simulink model "MagLevTbx_MagSens_v43_Block"  (R2025b)
settings: Solver=FixedStepDiscrete  StartTime=0.0  StopTime=Inf  FixedStep=0.05  RelTol=1e-3  EnableMultiTasking=on
settings Model: ExtModeTrigDuration=2  Creator=riccardo  LastModifiedBy=riccardo
settings SolverCC: AutoInsertRateTranBlk=on
settings OptimizationCC: EnhancedBackFolding=on  PassReuseOutputArgsAs=Individual arguments  ZeroExternalMemoryAtStartup=off  ZeroInternalMemoryAtStartup=off  MaxStackSize=64  OptimizeBlockOrder=speed  DifferentSizesBufferReuse=on  OptimizationCustomize=off  EfficientTunableParamExpr=on
settings DebuggingCC: ParameterTunabilityLossMsg=error
settings HardwareCC: ProdBitPerPointer=32.0  ProdBitPerSizeT=32.0  ProdBitPerPtrDiffT=32.0  ProdLargestAtomicInteger=Long  ProdLargestAtomicFloat=Double  ProdWordSize=32.0  ProdHWDeviceType=ARM Compatible->ARM Cortex
settings SFSimCC: MATLABDynamicMemAlloc=off
settings RTWCC: SystemTargetFile=ert.tlc  HardwareBoard=Teensy 4.1 (Arduino Compatible)  TemplateMakefile=ert_default_tmf  Toolchain=Arduino ARM M7  BuildConfiguration=Faster Runs  Description=Embedded Coder
settings CodeAppCC: ForceParamTrailComments=on  IgnoreCustomStorageClasses=off  OperatorAnnotations=on  SimulinkDataObjDesc=on  SFDataObjDesc=on  InsertBlockDesc=on
settings ERTTargetCC: ExtModeTransport=3.0  ExtModeStaticAlloc=on  ExtModeAutomaticAllocSize=off  ExtModeStaticAllocSize=65536.0  ExtModeMexFile=ext_xcp  ExtModeIntrfLevel=Level2 - Open  InlinedParameterPlacement=Hierarchical  RootIOFormat=Structure reference  TargetLangStandard=C99 (ISO)  SupportContinuousTime=on  SupportVariableSizeSignals=on

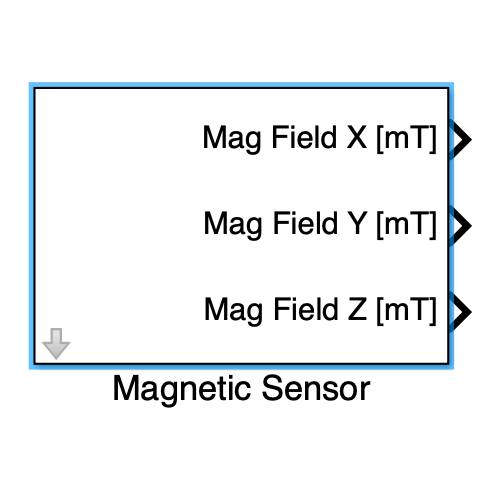
[thumbnail: Simulink's stored preview of the top-level diagram]
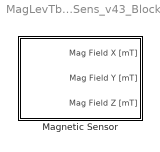
== system MagLevTbx_MagSens_v43_Block ==
  Magnetic Sensor : Subsystem  mask(Magnetic Sensor (Infineon TLV493D)){sampleTime=-1, showEnablePort=off}
      mask prompts: sampleTime "Sample time (-1 for inherited):"; showEnablePort "Show enable port"
      mask help: Get 3D magnetic field measurement (in [mT]) from the selected magnetic sensor.
      mask init:
      | MagLevTbx_MagSens_MaskInit(gcb, showEnablePort);
      mask Help:
      | Riccardo Antonello (riccardo.antonello@unipd.it)
      | 
      | February 17, 2026
      | 
      | Dept. of Information Engineering, University of Padova
      mask Callback sampleTime: MagLevTbx_MagSens_MaskCbFcn_SampleTime();

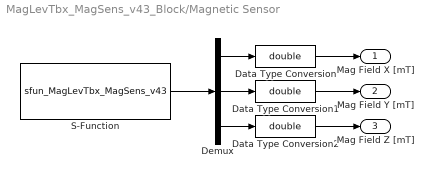
== system MagLevTbx_MagSens_v43_Block/Magnetic Sensor ==
  Data Type Conversion : DataTypeConversion  OutDataTypeStr=double  SaturateOnIntegerOverflow=off  RndMeth=Floor
  Data Type Conversion1 : DataTypeConversion  OutDataTypeStr=double  SaturateOnIntegerOverflow=off  RndMeth=Floor
  Data Type Conversion2 : DataTypeConversion  OutDataTypeStr=double  SaturateOnIntegerOverflow=off  RndMeth=Floor
  Demux : Demux  Outputs=3
  S-Function : S-Function  FunctionName=sfun_MagLevTbx_MagSens_v43  Parameters=sampleTime  SFunctionDeploymentMode=off  EnableBusSupport=off
  Mag Field X [mT] : Outport
  Mag Field Y [mT] : Outport  Port=2
  Mag Field Z [mT] : Outport  Port=3
  wires:
  Demux/3 -> Data Type Conversion2/1
  Demux/2 -> Data Type Conversion1/1
  Demux/1 -> Data Type Conversion/1
  S-Function/1 -> Demux/1
  Data Type Conversion/1 -> Mag Field X [mT]/1
  Data Type Conversion1/1 -> Mag Field Y [mT]/1
  Data Type Conversion2/1 -> Mag Field Z [mT]/1
